simulink model "model0"  (R2021a)
settings: Solver=FixedStepAuto  StartTime=0.0  StopTime=2  FixedStep=0.0001  RelTol=1e-3
libraries: pid_lib x1
settings Model: Creator=21694  LastModifiedBy=21694

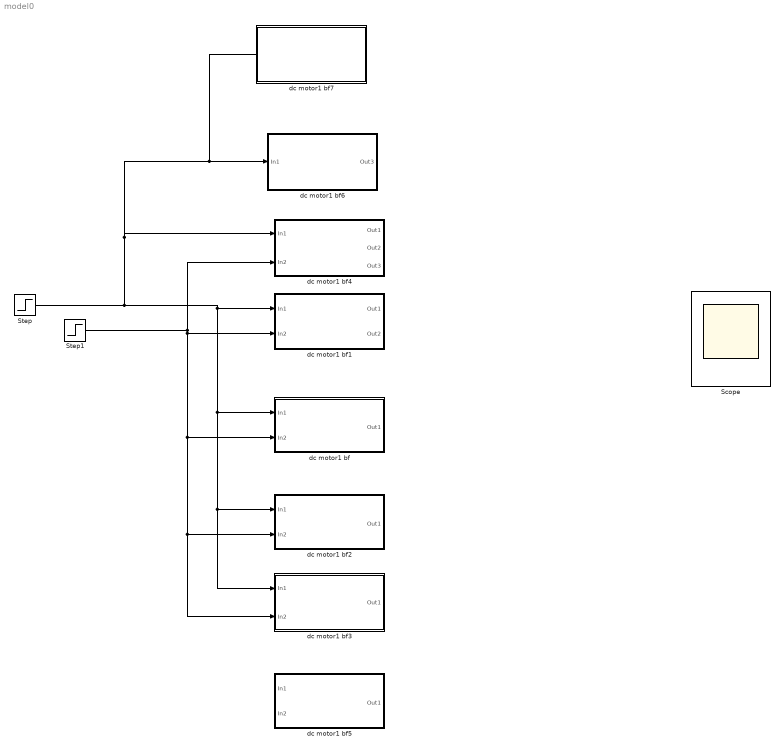
== system model0 ==
  Scope : Scope  NumInputPorts=2
  Step : Step  Time=0  After=100  SampleTime=0
  Step1 : Step  Time=0  After=0  SampleTime=0
  dc motor1 bf : Subsystem
  dc motor1 bf1 : Subsystem
  dc motor1 bf2 : Subsystem
  dc motor1 bf3 : Subsystem
  dc motor1 bf4 : Subsystem
  dc motor1 bf5 : Subsystem
  dc motor1 bf6 : Subsystem
  dc motor1 bf7 : Subsystem
  wires:
  Step/1 -> dc motor1 bf1/1(In1), dc motor1 bf2/1(In1), dc motor1 bf3/1(In1), dc motor1 bf/1(In1), dc motor1 bf4/1(In1), dc motor1 bf6/1(In1)
  Step1/1 -> dc motor1 bf4/2(In2), dc motor1 bf1/2(In2), dc motor1 bf2/2(In2), dc motor1 bf3/2(In2), dc motor1 bf/2(In2)
  ? -> Scope/1
  ? -> Scope/2

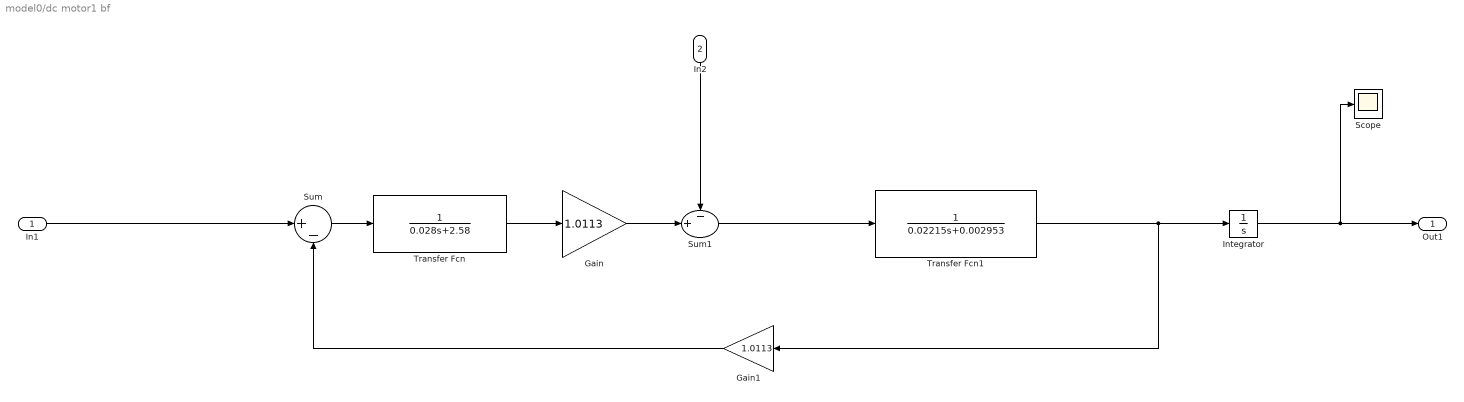
== system model0/dc motor1 bf ==
  In1 : Inport
  In2 : Inport  Port=2
  Gain : Gain  Gain=1.0113
  Gain1 : Gain  Gain=1.0113
  Integrator : Integrator  InitialCondition=3
  Scope : Scope
  Sum : Sum  Inputs=|+-
  Sum1 : Sum  Inputs=-+|
  Transfer Fcn : TransferFcn  Denominator=[0.028 2.58]
  Transfer Fcn1 : TransferFcn  Numerator=1  Denominator=[0.02215 0.002953]
  Out1 : Outport
  wires:
  Integrator/1 -> Scope/1, Out1/1
  In2/1 -> Sum1/1
  Transfer Fcn1/1 -> Integrator/1, Gain1/1
  Sum/1 -> Transfer Fcn/1
  Gain1/1 -> Sum/2
  Transfer Fcn/1 -> Gain/1
  Gain/1 -> Sum1/2
  Sum1/1 -> Transfer Fcn1/1
  In1/1 -> Sum/1

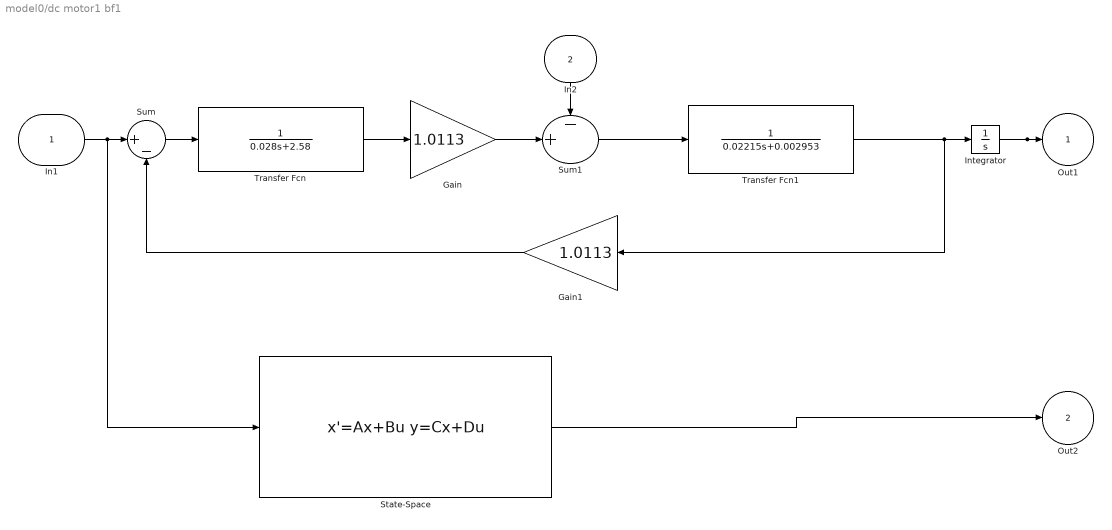
== system model0/dc motor1 bf1 ==
  In1 : Inport
  In2 : Inport  Port=2
  Gain : Gain  Gain=1.0113
  Gain1 : Gain  Gain=1.0113
  Integrator : Integrator
  State-Space : StateSpace  A=|  B=[35.7143;0;0]  C=[0 1 0]  D=0  InitialCondition=0
      | [-92.1429 0 -36.1179
      |  ;0 0 1.0000;
      | 45.6569   0   -0.1333]
  Sum : Sum  Inputs=|+-
  Sum1 : Sum  Inputs=-+|
  Transfer Fcn : TransferFcn  Denominator=[0.028 2.58]
  Transfer Fcn1 : TransferFcn  Numerator=1  Denominator=[0.02215 0.002953]
  Out1 : Outport
  Out2 : Outport  Port=2
  wires:
  In1/1 -> State-Space/1, Sum/1
  Sum1/1 -> Transfer Fcn1/1
  Gain/1 -> Sum1/2
  Transfer Fcn/1 -> Gain/1
  Gain1/1 -> Sum/2
  Sum/1 -> Transfer Fcn/1
  Transfer Fcn1/1 -> Integrator/1, Gain1/1
  In2/1 -> Sum1/1
  State-Space/1 -> Out2/1
  Integrator/1 -> Out1/1

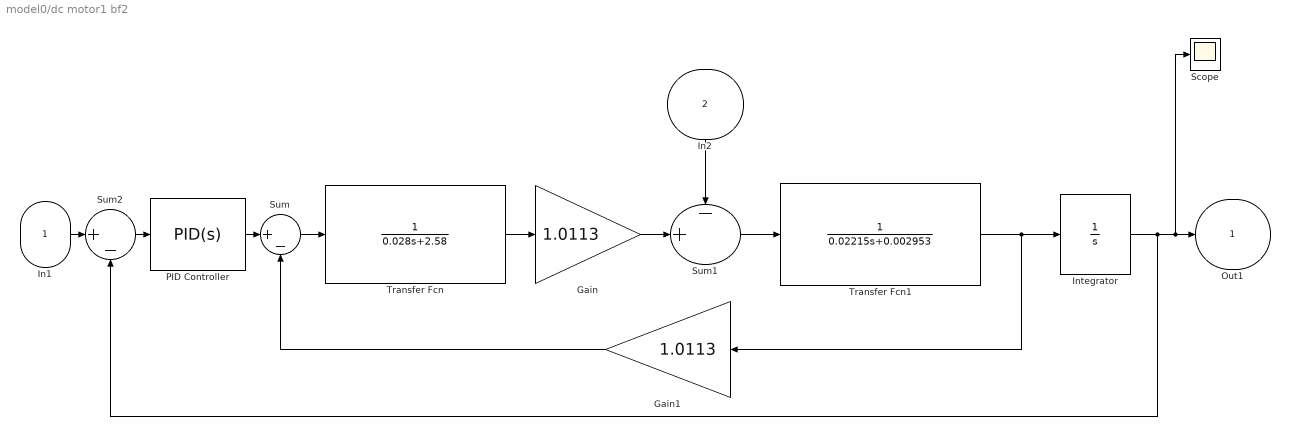
== system model0/dc motor1 bf2 ==
  In1 : Inport
  In2 : Inport  Port=2
  Gain : Gain  Gain=1.0113
  Gain1 : Gain  Gain=1.0113
  Integrator : Integrator  InitialCondition=3
  PID Controller : pid_lib/PID Controller  Controller=PID  Form=Parallel  TimeDomain=Continuous-time  UseExternalTs=off  SampleTime=-1  IntegratorMethod=Forward Euler  FilterMethod=Forward Euler  ControllerParametersSource=internal  P=1  I=0  D=0  UseFilter=on  N=100  TunerSelectOption=Transfer Function Based (PID Tuner App)  InitialConditionSource=internal  InitialConditionForIntegrator=0  InitialConditionForFilter=0  DifferentiatorICPrevScaledInput=0  ExternalReset=none  TrackingMode=off  Kt=1  LimitOutput=off  SatLimitsSource=internal  UpperSaturationLimit=inf  LowerSaturationLimit=-inf  LinearizeAsGain=on  AntiWindupMode=none  Kb=1  POutMin=[]  POutMax=[]  IOutMin=[]  IOutMax=[]  DOutMin=[]  DOutMax=[]  NOutMin=[]  NOutMax=[]  SumOutMin=[]  SumOutMax=[]  SaturationOutMin=[]  SaturationOutMax=[]  PParamMin=[]  PParamMax=[]  IParamMin=[]  IParamMax=[]  DParamMin=[]  DParamMax=[]  NParamMin=[]  NParamMax=[]  KbParamMin=[]  KbParamMax=[]  KtParamMin=[]  KtParamMax=[]  KbOutMin=[]  KbOutMax=[]  KtOutMin=[]  KtOutMax=[]  IntegratorOutMin=[]  IntegratorOutMax=[]  FilterOutMin=[]  FilterOutMax=[]  SumI1OutMin=[]  SumI1OutMax=[]  SumI2OutMin=[]  SumI2OutMax=[]  SumI3OutMin=[]  SumI3OutMax=[]  SumI4OutMin=[]  SumI4OutMax=[]  SumDOutMin=[]  SumDOutMax=[]  DifferentiatorOutMin=[]  DifferentiatorOutMax=[]  FilterDiffOutCoefMin=[]  FilterDiffOutCoefMax=[]  ReciprocalOutMin=[]  ReciprocalOutMax=[]  SumDenOutMin=[]  SumDenOutMax=[]  SumNumOutMin=[]  SumNumOutMax=[]  DivideOutMin=[]  DivideOutMax=[]  UdiffTsProdOutMin=[]  UdiffTsProdOutMax=[]  NTsProdOutMin=[]  NTsProdOutMax=[]  UintegralTsProdOutMin=[]  UintegralTsProdOutMax=[]  UngainTsProdOutMin=[]  UngainTsProdOutMax=[]  IntegratorContinuousStateAttributes=''  IntegratorStateMustResolveToSignalObject=off  IntegratorRTWStateStorageClass=Auto  FilterContinuousStateAttributes=''  FilterStateMustResolveToSignalObject=off  FilterRTWStateStorageClass=Auto  ParallelPVariant=InternalParameters  IdealPVariant=Disabled  IVariant=InternalParameters  DVariant=InternalParameters  IntegratorVariant=Continuous  SatVariant=Disabled  AWVariant=Passthrough  PCopyVariant=Disabled  TRVariant=Disabled  FdbkBlocksVariant=Forward  IdealPFdbkVariant=Disabled  SatFdbkVariant=Disabled  DerivativeFilterVariant=ContFilter  NVariant=InternalParameters  NCopyVariant=Disabled  FilterICVariant=InternalICsFilter  IntegratorICVariant=InternalICs  ExternalResetVariant=Disabled  TRSumVariant=Passthrough  SumFdbkVariant=Disabled  SumVariant=Sum_PID  TsampFilterVariant=InternalTs  TsampNgainVariant=Passthrough  TsampIntegralVariant=Passthrough  ExternalSaturationOutDataTypeStr=Inherit: Same as second input
  Scope : Scope
  Sum : Sum  Inputs=|+-
  Sum1 : Sum  Inputs=-+|
  Sum2 : Sum  Inputs=|+-
  Transfer Fcn : TransferFcn  Denominator=[0.028 2.58]
  Transfer Fcn1 : TransferFcn  Numerator=1  Denominator=[0.02215 0.002953]
  Out1 : Outport
  wires:
  In1/1 -> Sum2/1
  Sum1/1 -> Transfer Fcn1/1
  Gain/1 -> Sum1/2
  Transfer Fcn/1 -> Gain/1
  Gain1/1 -> Sum/2
  Sum/1 -> Transfer Fcn/1
  Transfer Fcn1/1 -> Integrator/1, Gain1/1
  In2/1 -> Sum1/1
  Integrator/1 -> Scope/1, Out1/1, Sum2/2
  Sum2/1 -> PID Controller/1
  PID Controller/1 -> Sum/1

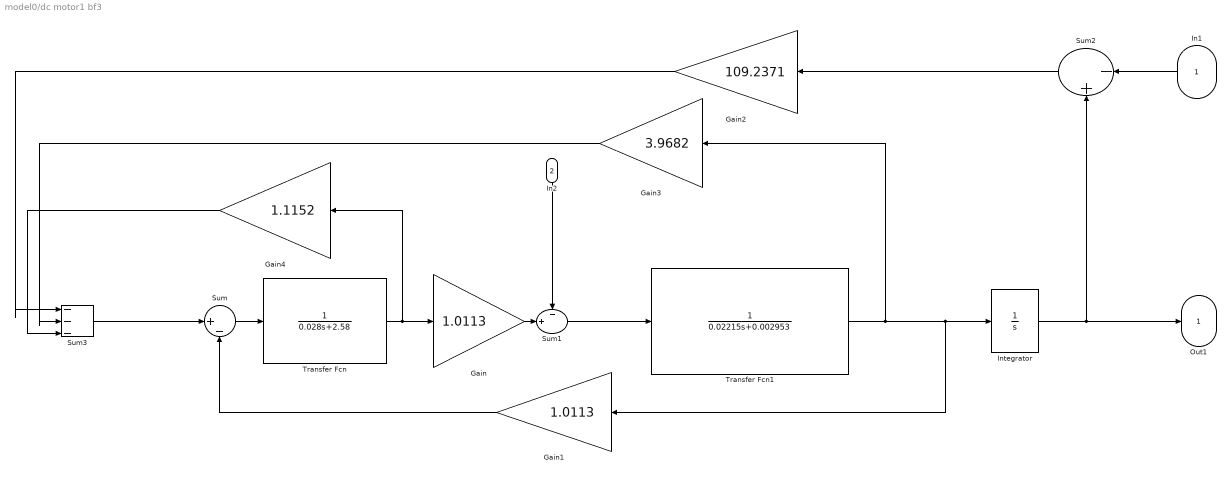
== system model0/dc motor1 bf3 ==
  In1 : Inport
  In2 : Inport  Port=2
  Gain : Gain  Gain=1.0113
  Gain1 : Gain  Gain=1.0113
  Gain2 : Gain  Gain=109.2371
  Gain3 : Gain  Gain=3.9682
  Gain4 : Gain  Gain=1.1152
  Integrator : Integrator  InitialCondition=3
  Sum : Sum  Inputs=|+-
  Sum1 : Sum  Inputs=-+|
  Sum2 : Sum  Inputs=|-+
  Sum3 : Sum  Inputs=|---
  Transfer Fcn : TransferFcn  Denominator=[0.028 2.58]
  Transfer Fcn1 : TransferFcn  Numerator=1  Denominator=[0.02215 0.002953]
  Out1 : Outport
  wires:
  Integrator/1 -> Sum2/2, Out1/1
  In2/1 -> Sum1/1
  Transfer Fcn1/1 -> Gain3/1, Integrator/1, Gain1/1
  Sum/1 -> Transfer Fcn/1
  Gain1/1 -> Sum/2
  Transfer Fcn/1 -> Gain4/1, Gain/1
  Gain/1 -> Sum1/2
  Sum1/1 -> Transfer Fcn1/1
  In1/1 -> Sum2/1
  Sum2/1 -> Gain2/1
  Gain2/1 -> Sum3/1
  Gain3/1 -> Sum3/2
  Gain4/1 -> Sum3/3
  Sum3/1 -> Sum/1

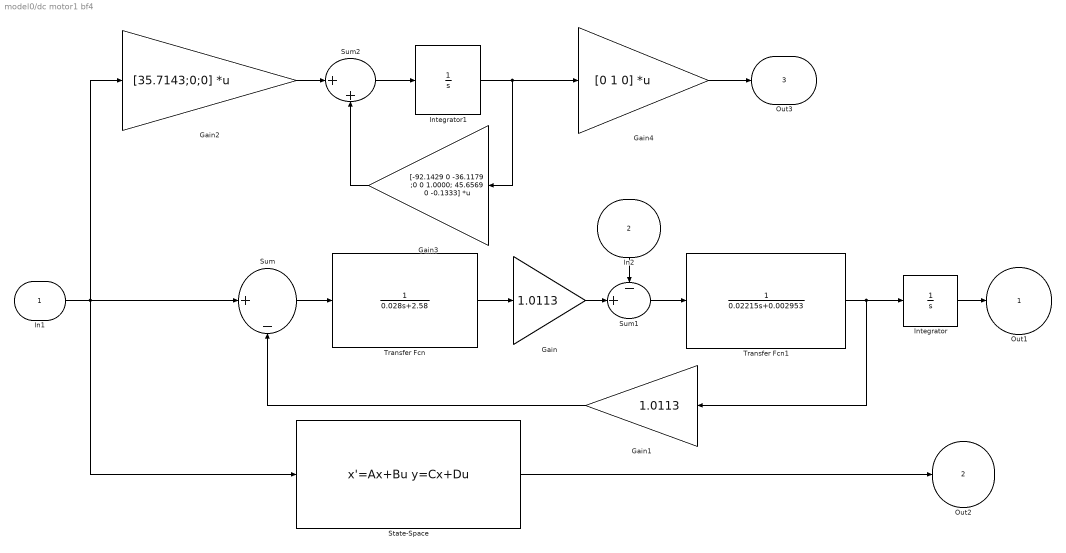
== system model0/dc motor1 bf4 ==
  In1 : Inport
  In2 : Inport  Port=2
  Gain : Gain  Gain=1.0113
  Gain1 : Gain  Gain=1.0113
  Gain2 : Gain  Gain=[35.7143;0;0]  Multiplication=Matrix(K*u)
  Gain3 : Gain  Gain=|  Multiplication=Matrix(K*u)
      | [-92.1429 0 -36.1179
      |  ;0 0 1.0000;
      | 45.6569   0   -0.1333]
  Gain4 : Gain  Gain=[0 1 0]  Multiplication=Matrix(K*u)
  Integrator : Integrator
  Integrator1 : Integrator
  State-Space : StateSpace  A=|  B=[35.7143;0;0]  C=[0 1 0]  D=0  InitialCondition=0
      | [-92.1429 0 -36.1179
      |  ;0 0 1.0000;
      | 45.6569   0   -0.1333]
  Sum : Sum  Inputs=|+-
  Sum1 : Sum  Inputs=-+|
  Sum2 : Sum  Inputs=|++
  Transfer Fcn : TransferFcn  Denominator=[0.028 2.58]
  Transfer Fcn1 : TransferFcn  Numerator=1  Denominator=[0.02215 0.002953]
  Out1 : Outport
  Out2 : Outport  Port=2
  Out3 : Outport  Port=3
  wires:
  State-Space/1 -> Out2/1
  In2/1 -> Sum1/1
  Transfer Fcn1/1 -> Integrator/1, Gain1/1
  Sum/1 -> Transfer Fcn/1
  Gain1/1 -> Sum/2
  Transfer Fcn/1 -> Gain/1
  Gain/1 -> Sum1/2
  Sum1/1 -> Transfer Fcn1/1
  In1/1 -> State-Space/1, Sum/1, Gain2/1
  Gain2/1 -> Sum2/1
  Sum2/1 -> Integrator1/1
  Gain4/1 -> Out3/1
  Integrator1/1 -> Gain3/1, Gain4/1
  Gain3/1 -> Sum2/2
  Integrator/1 -> Out1/1

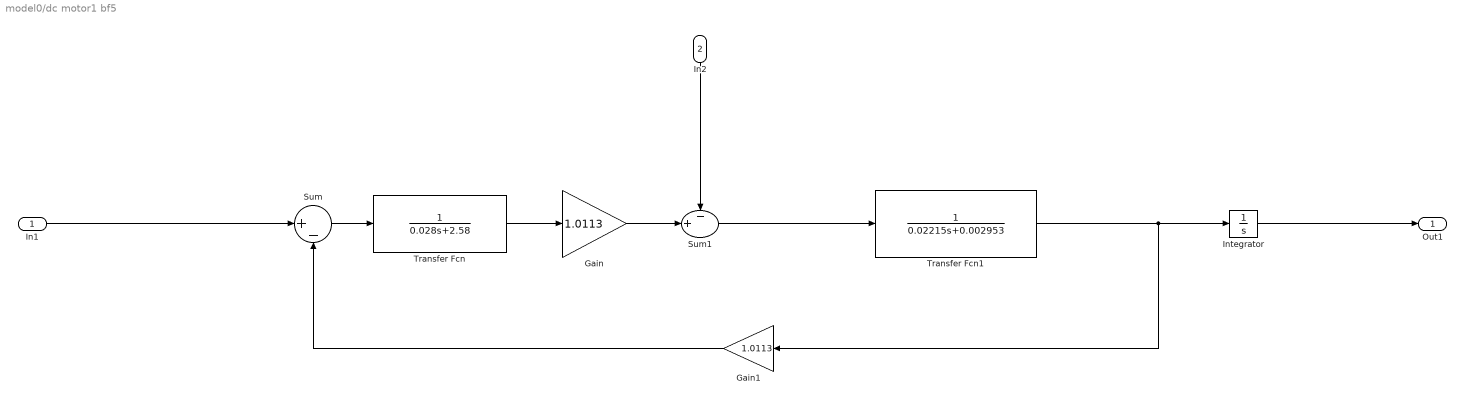
== system model0/dc motor1 bf5 ==
  In1 : Inport
  In2 : Inport  Port=2
  Gain : Gain  Gain=1.0113
  Gain1 : Gain  Gain=1.0113
  Integrator : Integrator  InitialCondition=3
  Sum : Sum  Inputs=|+-
  Sum1 : Sum  Inputs=-+|
  Transfer Fcn : TransferFcn  Denominator=[0.028 2.58]
  Transfer Fcn1 : TransferFcn  Numerator=1  Denominator=[0.02215 0.002953]
  Out1 : Outport
  wires:
  In1/1 -> Sum/1
  Sum1/1 -> Transfer Fcn1/1
  Gain/1 -> Sum1/2
  Transfer Fcn/1 -> Gain/1
  Gain1/1 -> Sum/2
  Sum/1 -> Transfer Fcn/1
  Transfer Fcn1/1 -> Gain1/1, Integrator/1
  In2/1 -> Sum1/1
  Integrator/1 -> Out1/1

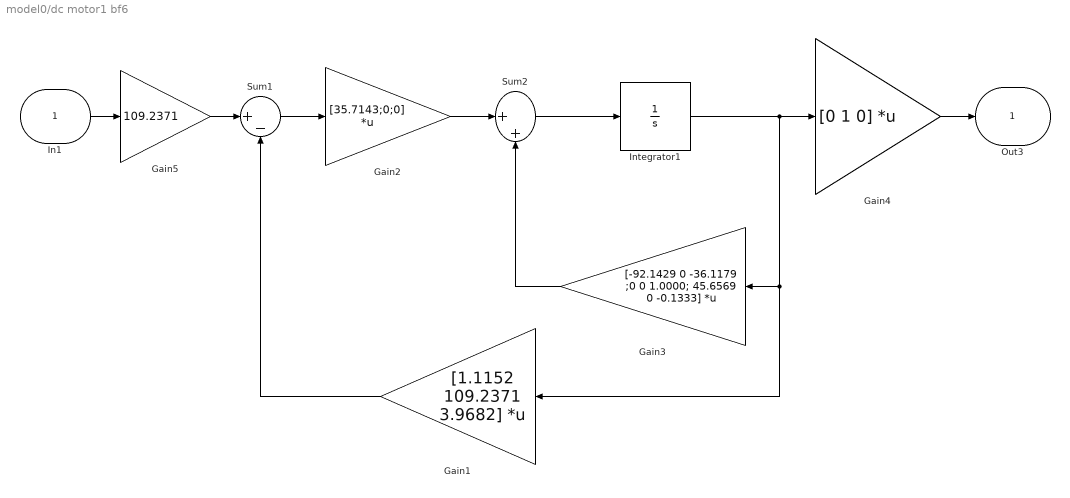
== system model0/dc motor1 bf6 ==
  In1 : Inport
  Gain1 : Gain  Gain="[1.1152  109.2371    3.9682]"  Multiplication=Matrix(K*u)
  Gain2 : Gain  Gain=[35.7143;0;0]  Multiplication=Matrix(K*u)
  Gain3 : Gain  Gain=|  Multiplication=Matrix(K*u)
      | [-92.1429 0 -36.1179
      |  ;0 0 1.0000;
      | 45.6569   0   -0.1333]
  Gain4 : Gain  Gain=[0 1 0]  Multiplication=Matrix(K*u)
  Gain5 : Gain  Gain=109.2371
  Integrator1 : Integrator
  Sum1 : Sum  Inputs=|+-
  Sum2 : Sum  Inputs=|++
  Out3 : Outport
  wires:
  Gain3/1 -> Sum2/2
  Integrator1/1 -> Gain1/1, Gain3/1, Gain4/1
  Gain4/1 -> Out3/1
  Sum2/1 -> Integrator1/1
  Gain2/1 -> Sum2/1
  In1/1 -> Gain5/1
  Gain1/1 -> Sum1/2
  Sum1/1 -> Gain2/1
  Gain5/1 -> Sum1/1

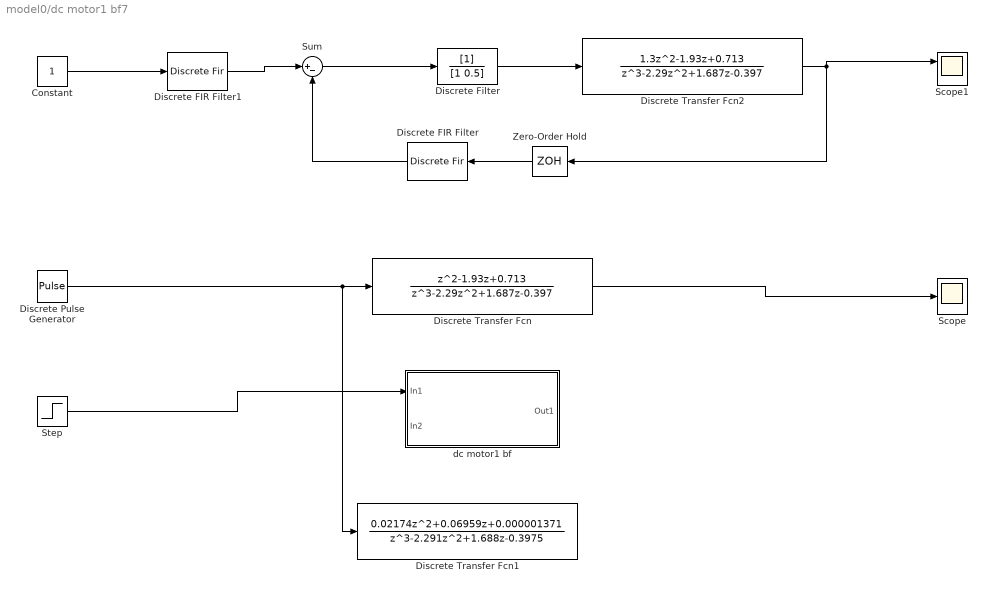
== system model0/dc motor1 bf7 ==
  Constant : Constant
  Discrete Pulse Generator : DiscretePulseGenerator  PulseType=Time based  Period=0.01  PulseWidth=5
  Discrete Transfer Fcn : DiscreteTransferFcn  Numerator=[1 -1.93 0.713]  Denominator=[1 -2.29 1.687 -0.397]
  Discrete Transfer Fcn1 : DiscreteTransferFcn  Numerator=[0.02174 0.06959 0.000001371]  Denominator="[1 -2.291 1.688  -0.3975]"
  Discrete Transfer Fcn2 : DiscreteTransferFcn  Numerator=[1.3 -1.93 0.713]  Denominator=[1 -2.29 1.687 -0.397]
  Discrete FIR Filter : DiscreteFir
  Discrete FIR Filter1 : DiscreteFir
  Discrete Filter : DiscreteFilter
  Scope : Scope
  Scope1 : Scope  NumInputPorts=2
  Step : Step  Time=0  SampleTime=0
  Sum : Sum  Inputs=|+-
  Zero-Order Hold : ZeroOrderHold  SampleTime=-1
  dc motor1 bf : Subsystem
  wires:
  Discrete Pulse Generator/1 -> Discrete Transfer Fcn1/1, Discrete Transfer Fcn/1
  Step/1 -> dc motor1 bf/1(In1)
  Constant/1 -> Discrete FIR Filter1/1
  Discrete FIR Filter1/1 -> Sum/1
  Sum/1 -> Discrete Filter/1
  Discrete Filter/1 -> Discrete Transfer Fcn2/1
  Zero-Order Hold/1 -> Discrete FIR Filter/1
  Discrete FIR Filter/1 -> Sum/2
  Discrete Transfer Fcn2/1 -> Zero-Order Hold/1, Scope1/1
  Discrete Transfer Fcn/1 -> Scope/1

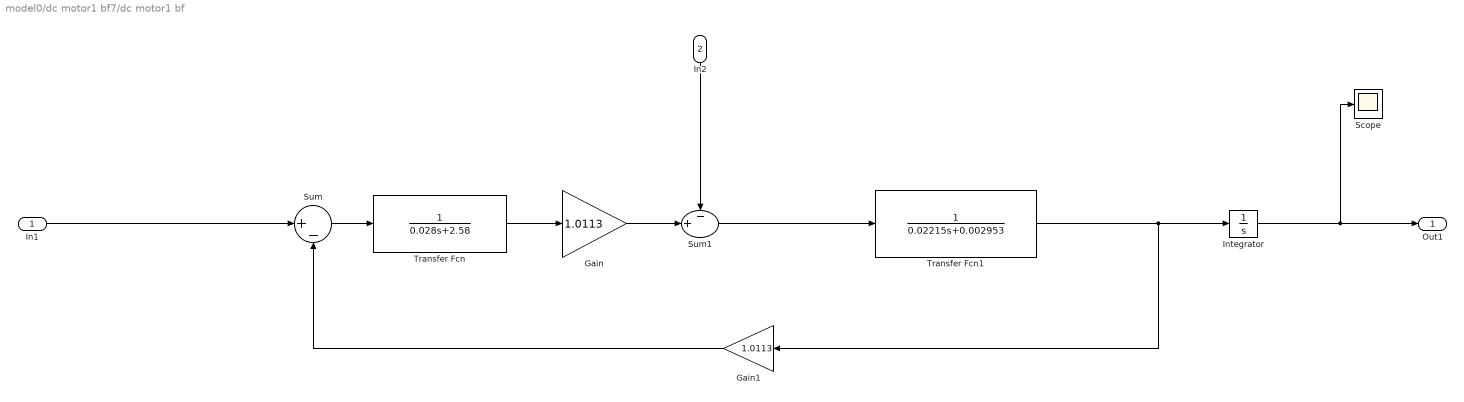
== system model0/dc motor1 bf7/dc motor1 bf ==
  In1 : Inport
  In2 : Inport  Port=2
  Gain : Gain  Gain=1.0113
  Gain1 : Gain  Gain=1.0113
  Integrator : Integrator
  Scope : Scope
  Sum : Sum  Inputs=|+-
  Sum1 : Sum  Inputs=-+|
  Transfer Fcn : TransferFcn  Denominator=[0.028 2.58]
  Transfer Fcn1 : TransferFcn  Numerator=1  Denominator=[0.02215 0.002953]
  Out1 : Outport
  wires:
  Integrator/1 -> Scope/1, Out1/1
  In2/1 -> Sum1/1
  Transfer Fcn1/1 -> Integrator/1, Gain1/1
  Sum/1 -> Transfer Fcn/1
  Gain1/1 -> Sum/2
  Transfer Fcn/1 -> Gain/1
  Gain/1 -> Sum1/2
  Sum1/1 -> Transfer Fcn1/1
  In1/1 -> Sum/1
